simulink model "LaneDetection"  (R2020b)
settings: Solver=VariableStepAuto  StartTime=0.0  StopTime=inf  RelTol=1e-3
libraries: dspvision x1, deeplib x1, visiongeotforms x1
settings Model: Creator=hmcl  LastModifiedBy=hmcl
settings OptimizationCC: ZeroExternalMemoryAtStartup=off  ZeroInternalMemoryAtStartup=off  InitFltsAndDblsToZero=on
settings HardwareCC: ProdLongLongMode=on  TargetLongLongMode=on
settings SFSimCC: SimTargetLang=C++  GPUAcceleration=on  SimDLTargetLibrary=cudnn
settings RTWCC: TargetLang=C++  GenerateGPUCode=CUDA  DLTargetLibrary=cudnn
settings GRTTargetCC: TargetLangStandard=C++03 (ISO)  CodeInterfacePackaging=C++ class

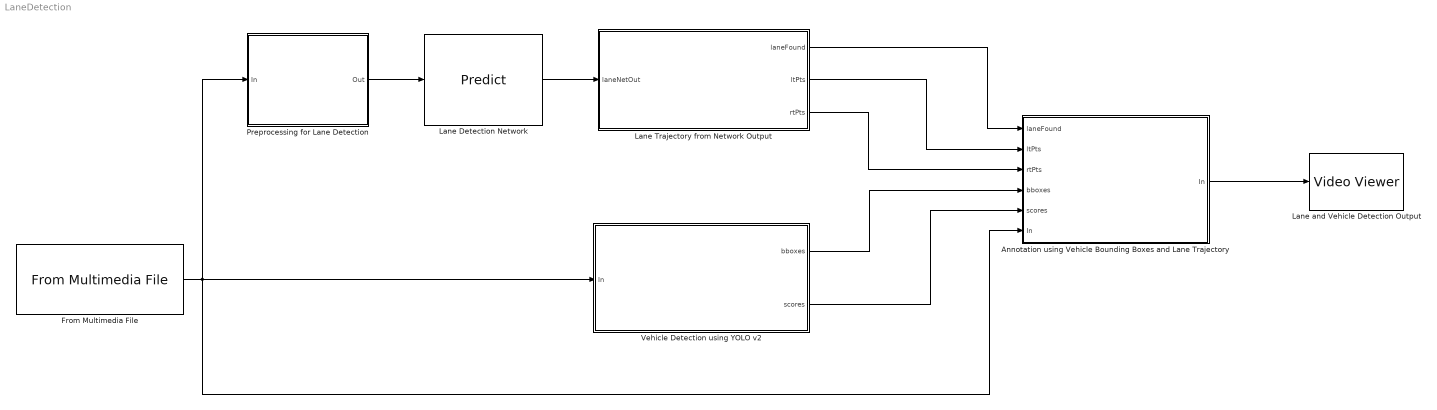
== system LaneDetection ==
  "Annotation using Vehicle Bounding Boxes and Lane Trajectory " : MATLAB Function  TreatAsAtomicUnit=on
  From Multimedia File : dspvision/From Multimedia File  inputFilename=/home/hmcl/ADcontrol/caltech_washington1.avi  readRange=[1 Inf]  loop=on  numPlays=inf  outputStreams=Video only  videoDataType=single  audioDataType=double  inheritSampleTime=on  userDefinedSampleTime=1/30  noAudioOutput=off  isIntensityVideo=off  fourcc=RGB  colorVideoFormat=One multidimensional signal  outputEOF=off  dataOrg=Column-major  audioFrameSize=1024  computeAudioFrameSize=off  outSamplingMode=Sample based
  Lane Detection Network : deeplib/Predict  Network=Network from MAT-file  NetworkFunction=squeezenet  NetworkFilePath=trainedLaneNet.mat  MiniBatchSize=128  InputDataFormats={ '', '' }  Predictions=on  Activations={}  ForceInterpretedSim=off  EnableDLNetwork=off
      settings: SourceProductBaseCode=NN
  "Lane Trajectory from Network Output " : MATLAB Function  TreatAsAtomicUnit=on
  Lane and Vehicle Detection Output : VideoViewer  FigPos=[74 892 644 507]
  Preprocessing for Lane Detection : Subsystem  TreatAsAtomicUnit=on
  Vehicle Detection using YOLO v2 : MATLAB Function  TreatAsAtomicUnit=on
  wires:
  Preprocessing for Lane Detection/1(Out) -> Lane Detection Network/1
  Vehicle Detection using YOLO v2/2(scores) -> "Annotation using Vehicle Bounding Boxes and Lane Trajectory "/5(scores)
  "Annotation using Vehicle Bounding Boxes and Lane Trajectory "/1(In) -> Lane and Vehicle Detection Output/1
  Lane Detection Network/1 -> "Lane Trajectory from Network Output "/1(laneNetOut)
  From Multimedia File/1 -> Preprocessing for Lane Detection/1(In), Vehicle Detection using YOLO v2/1(In), "Annotation using Vehicle Bounding Boxes and Lane Trajectory "/6("In ")
  "Lane Trajectory from Network Output "/2(ltPts) -> "Annotation using Vehicle Bounding Boxes and Lane Trajectory "/2(ltPts)
  "Lane Trajectory from Network Output "/3(rtPts) -> "Annotation using Vehicle Bounding Boxes and Lane Trajectory "/3(rtPts)
  Vehicle Detection using YOLO v2/1(bboxes) -> "Annotation using Vehicle Bounding Boxes and Lane Trajectory "/4(bboxes)
  "Lane Trajectory from Network Output "/1(laneFound) -> "Annotation using Vehicle Bounding Boxes and Lane Trajectory "/1(laneFound)

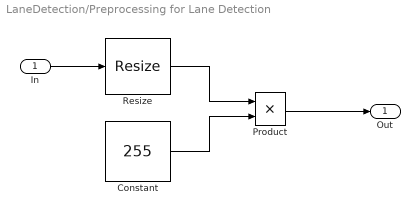
== system LaneDetection/Preprocessing for Lane Detection ==
  In : Inport
  Constant : Constant  Value=255
  Product : Product
  Resize : visiongeotforms/Resize  specify=Number of output rows and columns  rfactor=[200 150]  outCols=25  outRows=25  outRowsCols=[227 227]  interp_method=Bilinear  antialias=on  useROI=off  roiFlag=off  roundingMode=Nearest  overflowMode=on  prodOutputMode=Binary point scaling  prodOutputWordLength=32  prodOutputFracLength=10
      settings: SourceProductBaseCode=VP
  Out : Outport
  wires:
  Constant/1 -> Product/2
  Resize/1 -> Product/1
  In/1 -> Resize/1
  Product/1 -> Out/1

== matlab function LaneDetection/Lane Trajectory from Network Output  ==
  data: laneNetOut input; laneFound output; ltPts output; rtPts output
function [laneFound,ltPts,rtPts] = LaneDetectionCoordinates(laneNetOut)

[laneFound,ltPts,rtPts] = lane_detection_coordinates(laneNetOut);

end

== matlab function LaneDetection/Annotation using Vehicle Bounding Boxes and Lane Trajectory  ==
  data: laneFound input; ltPts input; rtPts input; bboxes input size=[20 4]; scores input size=[20  1]; In input; In output
function In = LaneVehicleAnnotation(laneFound, ltPts, rtPts, bboxes, scores, In)

In = lane_vehicle_annotation(laneFound, ltPts, rtPts, bboxes, scores, In);

end

== matlab function LaneDetection/Vehicle Detection using YOLO v2 ==
  data: bboxes output size=[20 4] [..100000]; In input; scores output size=[20 1]
function [bboxes,scores] = VehicleDetectionYOLOv2(In)

[bboxes,scores] = vehicle_detection_yolo_v2(In);

end
